simulink library "etherlab_lib"  (Simulink 7.4)
settings: Solver=ode45  SolverMode=SingleTasking  StartTime=0.0  StopTime=10.0  RelTol=1e-3
undefined symbols (not defined in the file or in its folder): Address, baumer_ecatencoder, el320x, el500x, el5101, el5101_0010, EL5151, El5152, el515x, ep41xx, ep43xx, rv, x
(part 1 of 3)
settings Model: Creator=rich  LastModifiedBy=ha  ExtModeAutoUpdateStatusClock=off

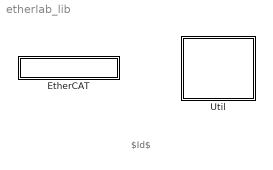
== system etherlab_lib ==
  note: $Id$
  EtherCAT : Subsystem
      mask Display: image(imread('ethercat_mini.png'))
  Util : Subsystem
      mask Display: image(imread('tools.png'))

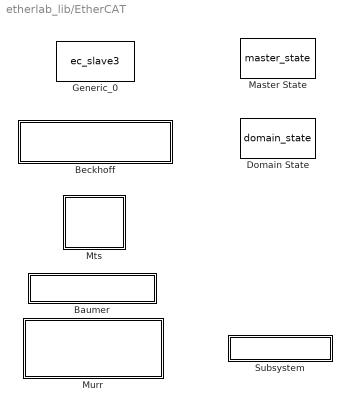
== system etherlab_lib/EtherCAT ==
  Baumer : Subsystem
      mask Display: image(imread('Baumer.png'))
  Beckhoff : Subsystem
      mask Display: image(imread('Beckhoff.png'))
  Domain State : S-Function  FunctionName=domain_state  Parameters=master,domain,input,output,io_domain,tsample  SFunctionModules='ecrt_support'  EnableBusSupport=off  mask(Domain State){master=0, domain=0, direction=Input and Output, io_domain=on, tsample=0}
      mask prompts: io_domain "Tx and RxPdo in one domain"; tsample "Sample Time"
      mask help:
      | Displays the following domain state information:
      | * Working Counter
      | * Domain state:
      | 	0 - No slaves
      | 	1 - Domain incomplete
      | 	2 - Domain complete
      mask init:
      | switch direction
      |     case 1
      |         input = 1;
      |         output = 0;
      |     case 2
      |         input = 0;
      |         output = 1;
      |     case 3
      |         input = 1;
      |         output = 1;
      | end
      mask StyleString: edit,edit,popup(Input Only|Output Only|Input and Output),checkbox,edit
      mask Display: fprintf('Domain State\nM:%u d:%u', master,domain);
  Generic_0 : S-Function  FunctionName=ec_slave3  Parameters=Address,rv.SlaveConfig,rv.PortConfig,debug,tsample  SFunctionModules='ecrt_support'  EnableBusSupport=off  mask(Generic EtherCAT Slave){master=0, index=1, rv=[], tsample=0, debug=0}
      mask prompts: index "Slave Index"; rv "EtherCAT Slave Configuration struct. (SlaveConfig, PortConfig)"; tsample "Sample Time"
      mask help:
      | The generic EtherCAT Slave is used to create any slave not contained
      | in this library. A mask input variable, <b>EtherCAT Slave Configuration</b>,
      | has to be set up by the user. This configures the slave.
      mask init:
      | masterStr = '';
      | positionStr = '';
      | 
      | [Address masterStr positionStr] = ...
      |     getEtherCATAddress(gcb,master,index,tsample);
      | 
      | 
      | if ~isfield(rv,'PortConfig') || isempty(rv)
      |    rv.PortConfig = [];
      | end
      | 
      | if ~isfield(rv,'SlaveConfig') || isempty(rv)
      |    rv.SlaveConfig = [];
      | end
      | 
      | if ~isfield(rv.SlaveConfig,'description') || isempty(rv)
      |    slave_name = 'unknown';
      | else
      |    slave_name = rv.SlaveConfig.description;
      | end
      mask Help: web(etherlab_help_path('generic.html'), '-helpbrowser');
      mask Display:
      | fprintf('Generic Slave\n%s \n%s Idx:%s',...
      |     slave_name, masterStr, positionStr)
  Master State : S-Function  FunctionName=master_state  Parameters=master,devices,reset,sync_dec,tsample  SFunctionModules='ecrt_support'  EnableBusSupport=off  mask(Master State){master=0, devices=1, reset=off, sync_dec=0, tsample=0}
      mask prompts: devices "Device Count"; reset "Reset Port"; sync_dec "Reference Clock Sync Decimation"; tsample "Sample Time"
      mask help:
      | Outputs master state:
      | * number of responding slaves
      | * Slave states
      | * Link up
      |
      | Enabling <b>Master Reset</b> forces the master to reset the bus
      | and scan for new slaves
      mask Display: fprintf('Master State\nM: %u', master);
  Mts : Subsystem
      mask Display: image(imread('mts-logo.png'))
  Murr : Subsystem
      mask Display: image(imread('Murr.png'))
  Subsystem : Subsystem
      settings: OpenFcn=[];
      mask Display: image(imread('ethercat_mini.png'))

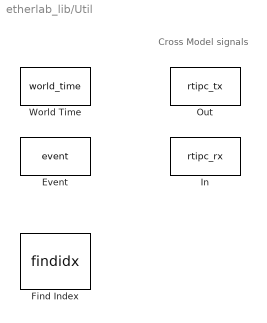
== system etherlab_lib/Util ==
  note: Cross Model signals
  Event : S-Function  FunctionName=event  Parameters=width,singleshot,dtype,tsample  EnableBusSupport=off  mask(Trigger Events){width=1, singleshot=on, dtype_str=Boolean, tsample=0}
      mask prompts: singleshot "Single shot"; dtype_str "Data Type"; tsample "Sample Time"
      mask help:
      | This block is used to generate an events on its output.
      |
      | Checking the "One Shot" option will generate only one event, otherwise a whole chain of events is generated for every count that the parameter value was incremented.
      mask init:
      | switch dtype_str
      |     case 'Unsigned Integer'
      |         dtype = 32;
      |     case 'Boolean'
      |         dtype = 1;
      |     otherwise
      |         dtype = 1;
      | end
      mask Help:
      | A typical problem with interactive constants, e.g. those that are connected to push buttons on the desktop, is that the events get lost due to it being set and reset too within one calculation cycle and thus is "lost".
      | 
      | This typically happens with push buttons acting on a constant. Sometimes the user presses and releases the push button so quickly that these separate events are send to the Real Time Application together as a single operation. The constant is then set and reset without the Application realising that there even was an event.
      | 
      | This block is overcomes this limitation by keeping an internal counter synchronised to a parameter value. If these two values are unequal, the output is toggled either:
      | * If the "Single Shot" option is checked, only one event pulse is generated and the internal counter is set to the parameter value.
      | * Without this option, the internal counter is incremented until it equals the parameter value, generating one event pulse for every increment.
      mask StyleString: edit,checkbox,popup(Boolean|Unsigned Integer),edit
      mask Display: disp('Event')
  Find Index : S-Function  FunctionName=findidx  Parameters=cmp,tsample  EnableBusSupport=off  mask(Find MinMax){cmp=First Minimum, tsample=-1}
      mask prompts: cmp "Comparison"; tsample "Sample Time"
      mask help:
      | This block takes a vector input and outputs:
      | 1: Found count
      | 2: Found Index (zero based)
      | 3: Value
      mask Help: This block finds the minimum or or maximum as well as the associated index from a vector of signals. The index is zero based.
      mask StyleString: popup(First Minimum|Last Minimum|First Maximum|Last Maximum),edit
      mask Display:
      | port_label('output',1,'Found');
      | port_label('output',2,'Index');
      | port_label('output',3,'Value');
  In : S-Function  FunctionName=rtipc_rx  Parameters=varname,dtype,len,force,tsample  SFunctionModules='rtipc'  EnableBusSupport=off  mask(Generic Output Port){varname='SIG01', dtype=double, len=1, force=off, tsample=0}
      mask prompts: varname "Signal Name"; dtype "Data Type"; len "Vector Length"; force "Enable value forcing"; tsample "Sample Time (-1 for inherited)"
      mask help:
      | RealTime Interprocess Communication input
      |
      | Signal Name: Name of signal to connect to (string)
      | Data Type: Signal's data type
      | Vector Length: Number of elements
      | Enable Force Value: Adds additional parameters to force the output value
      mask StyleString: edit,popup(boolean|int8|uint8|int16|uint16|int32|uint32|single|double),edit,checkbox,edit
      mask Display: fprintf(varname)
  Out : S-Function  FunctionName=rtipc_tx  Parameters=varname,force,tsample  SFunctionModules='rtipc'  EnableBusSupport=off  mask(Generic Output Port){varname='SIG01', force=off, tsample=-1}
      mask prompts: varname "Signal Name"; force "Enable value forcing"; tsample "Sample Time (-1 for inherited)"
      mask Display: fprintf(varname)
  World Time : S-Function  FunctionName=world_time  Parameters=tsample  EnableBusSupport=off  mask(World Time){tsample=0}
      mask prompts: tsample "Sample Time"
      mask help: Outputs the current world time for the given sample time.
      mask Help: This block outputs the hosts current real world time in seconds since 1.1.1970

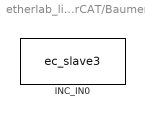
== system etherlab_lib/EtherCAT/Baumer ==
  INC_IN0 : S-Function  LoadFcn=baumer_ecatencoder('check');  FunctionName=ec_slave3  Parameters=Address,rv.SlaveConfig,rv.PortConfig,debug,tsample  SFunctionModules='ecrt_support'  EnableBusSupport=off  mask(Baumer && Thalheim ATD Encoder){master=0, index=1, model=BT ATD2_PoE, dcmode=DC on, dccustom=[ hex2dec('300') 0 0 0 0 0 0 0 0 0], direction=CW, tsample=0, debug=0}
      mask prompts: index "Slave Index"; model "Device Model"; dcmode "DC Mode"; dccustom "DC Customer"; direction "Counting direction"; tsample "Sample Time (-1 for inherited)"
      mask help: Baumer & Thalheim ATD Encoder
      mask init:
      | masterStr = '';
      | positionStr = '';
      | [Address masterStr positionStr] = ...
      |     getEtherCATAddress(gcb,master,index,tsample);
      | 
      | baumer_ecatencoder('set');
      | 
      | rv = get_param(gcbh,'UserData');
      | 
      | % Bit2 must be set, this is a firmware bug
      | rv.SlaveConfig.sdo = {hex2dec('6000'),0,16,(direction-1)+4};
      mask Help: web(etherlab_help_path('baumer-ecatencoder.html'), '-helpbrowser');
      mask StyleString: edit,edit,popup(BT ATD2|BT ATD2_PoE|BT ATD4),popup(DC off|DC on|DC Customized),edit,popup(CW|CCW),edit,edit
      mask CallbackString: |||baumer_ecatencoder('ui');||||
      mask Display: fprintf('%s\nM:%s Idx:%s',model,masterStr,positionStr)
